simulink model "control_loop_2006a"  (Simulink 7.7)
settings: Solver=ode45  StartTime=0.0  StopTime=1  RelTol=1e-10
values from neighbouring files (symbols this model uses):
  alpha = zeros(length(a),1)    [auto_tune_param_main_ovsInvestigation_typeI.m]
  kp_est = plant_loc.kp_est    [auto_tune_2ndOrder_calculate_overshoot_2.m]
  tp1 = plant_loc.tp1    [auto_tune_param_calculateOvs.m]    (also in auto_tune_param_calculateOvs_x_y.m; auto_tune_param_calculateOvs_x_y_margaris.m; auto_tune_param_mainTspEstimation.m; auto_tune_param_main_SettlingTimePlant.m)
  tp2 = plant_loc.tp2    [auto_tune_param_calculateOvs.m]    (also in auto_tune_param_calculateOvs_x_y.m; auto_tune_param_calculateOvs_x_y_margaris.m; auto_tune_param_mainTspEstimation.m; auto_tune_param_main_SettlingTimePlant.m)
  tp3 = plant_loc.tp3    [auto_tune_param_calculateOvs.m]    (also in auto_tune_param_calculateOvs_x_y.m; auto_tune_param_calculateOvs_x_y_margaris.m; auto_tune_param_mainTspEstimation.m; auto_tune_param_main_SettlingTimePlant.m)
libraries: cstblocks x13
settings Model: Creator=kostis  LastModifiedBy=kostis
settings OptimizationCC: InitFltsAndDblsToZero=on
settings DebuggingCC: SaveWithParameterizedLinksMsg=none  SignalResolutionControl=TryResolveAllWithWarning  MultiTaskDSMMsg=warning  MultiTaskCondExecSysMsg=none  StrictBusMsg=None
settings HardwareCC: TargetHWDeviceType=32-bit Generic
settings RTWCC: IncludeERTFirstTime=on
settings GRTTargetCC: TargetFcnLib=ansi_tfl_tmw.mat

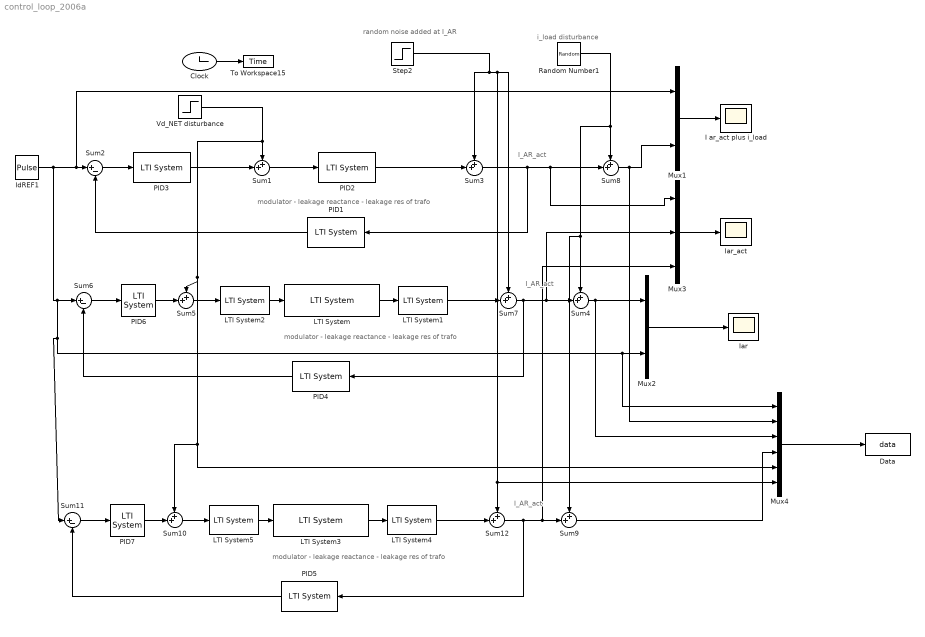
== system control_loop_2006a ==
  note: modulator - leakage reactance - leakage res of trafo
  note: i_load disturbance
  note: random noise added at I_AR
  note: modulator - leakage reactance - leakage res of trafo
  note: I_AR_act
  note: I_AR_act
  note: modulator - leakage reactance - leakage res of trafo
  note: I_AR_act
  Clock : Clock
      settings: Decimation=10
  Data : ToWorkspace  VariableName=data  SampleTime=-1  SaveFormat=Structure
  I ar_act plus i_load : Scope
      settings: TickLabels=on  TimeRange=40  YMin=-0.05  YMax=1.1  SaveName=OutputSignal1  SampleInput=on  SampleTime=0.001
  Iar : Scope
      settings: TickLabels=on  TimeRange=40  YMin=0  YMax=2  SaveName=OutputSignal  SampleInput=on  SampleTime=0.001
  Iar_act : Scope
      settings: TickLabels=on  TimeRange=40  YMin=0  YMax=2  SaveName=OutputSignal2  SampleInput=on  SampleTime=0.001
  IdREF1 : DiscretePulseGenerator  PulseType=Time based  Period=10  PulseWidth=50  PhaseDelay=0.35
  LTI System : cstblocks/LTI System  SystemSampleTime=-1  sys=tf(1,[tp1*tp3 tp1+tp3 1])  IC=[]
  LTI System1 : cstblocks/LTI System  SystemSampleTime=-1  sys=tf(1,[tp2 1])  IC=[]
  LTI System2 : cstblocks/LTI System  SystemSampleTime=-1  sys=tf(kp_est*(1+alpha),1)  IC=[]
  LTI System3 : cstblocks/LTI System  SystemSampleTime=-1  sys=tf(1,[tp1*tp3 tp1+tp3 1])  IC=[]
  LTI System4 : cstblocks/LTI System  SystemSampleTime=-1  sys=tf(1,[tp2 1])  IC=[]
  LTI System5 : cstblocks/LTI System  SystemSampleTime=-1  sys=tf(kp_est*(1-alpha),1)  IC=[]
  Mux1 : Mux  Inputs=2
  Mux2 : Mux  Inputs=2
  Mux3 : Mux  Inputs=3
  Mux4 : Mux  Inputs=6
  PID1 : cstblocks/LTI System  SystemSampleTime=-1  sys=kh  IC=[]
  PID2 : cstblocks/LTI System  SystemSampleTime=-1  sys=Gp  IC=[]
  PID3 : cstblocks/LTI System  SystemSampleTime=-1  sys=Gc  IC=[]
  PID4 : cstblocks/LTI System  SystemSampleTime=-1  sys=kh  IC=[]
  PID5 : cstblocks/LTI System  SystemSampleTime=-1  sys=kh  IC=[]
  PID6 : cstblocks/LTI System  SystemSampleTime=-1  sys=Gc  IC=[]
  PID7 : cstblocks/LTI System  SystemSampleTime=-1  sys=Gc  IC=[]
  Random Number1 : RandomNumber  Variance=0.00005  Seed=0.025  SampleTime=0.0001
  Step2 : Step  Time=0.75  After=0.7  SampleTime=0
  Sum{1,3..5,7..10,12} (9 alike) : Sum  Inputs=++|
  Sum11 : Sum  Inputs=|+-
  Sum2 : Sum  Inputs=|+-
  Sum6 : Sum  Inputs=|+-
  To Workspace15 : ToWorkspace  VariableName=Time  SampleTime=-1  SaveFormat=Array
  Vd_NET disturbance : Step  Time=0.5  After=0.8  SampleTime=0
  wires:
  PID3/1 -> Sum1/2
  Sum1/1 -> PID2/1
  Vd_NET disturbance/1 -> Sum1/1, Sum5/1, Mux4/5, Sum10/1
  Sum2/1 -> PID3/1
  PID1/1 -> Sum2/2
  PID2/1 -> Sum3/2
  Sum3/1 -> PID1/1, Sum8/2, Mux3/1
  IdREF1/1 -> Sum6/1, Sum11/1, Mux2/2, Mux4/1, Sum2/1, Mux1/1
  PID6/1 -> Sum5/2
  Sum6/1 -> PID6/1
  PID4/1 -> Sum6/2
  Sum7/1 -> PID4/1, Sum4/2, Mux3/2
  LTI System1/1 -> Sum7/2
  LTI System/1 -> LTI System1/1
  Sum5/1 -> LTI System2/1
  LTI System2/1 -> LTI System/1
  Step2/1 -> Sum3/1, Sum7/1, Mux4/6, Sum12/1
  Random Number1/1 -> Sum8/1, Sum4/1, Sum9/1
  Sum4/1 -> Mux2/1, Mux4/3
  Mux2/1 -> Iar/1
  Mux1/1 -> I ar_act plus i_load/1
  Mux3/1 -> Iar_act/1
  Sum8/1 -> Mux1/2, Mux4/2
  Mux4/1 -> Data/1
  PID7/1 -> Sum10/2
  Sum11/1 -> PID7/1
  PID5/1 -> Sum11/2
  Sum12/1 -> PID5/1, Sum9/2, Mux3/3
  LTI System4/1 -> Sum12/2
  LTI System3/1 -> LTI System4/1
  Sum10/1 -> LTI System5/1
  LTI System5/1 -> LTI System3/1
  Sum9/1 -> Mux4/4
  Clock/1 -> To Workspace15/1
